simulink model "Tank1"  (R2023a)
settings: Solver=VariableStepAuto  StartTime=0.0  StopTime=100  RelTol=1e-3
settings Model: Creator=hch  LastModifiedBy=hch

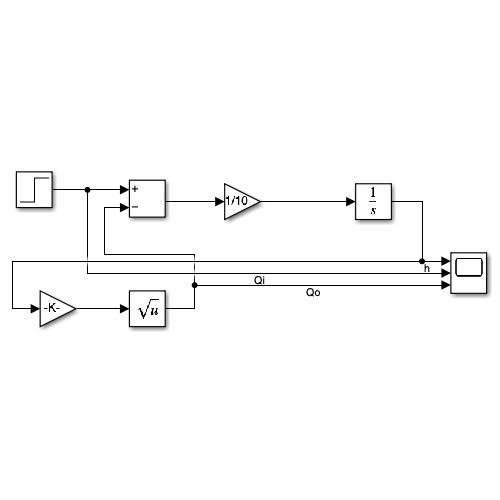
[thumbnail: Simulink's stored preview of the top-level diagram]
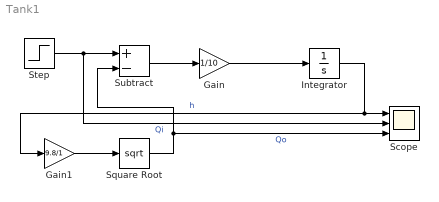
== system Tank1 ==
  Gain : Gain  Gain=1/10
  Gain1 : Gain  Gain=9.8/1
  Integrator : Integrator  InitialCondition=10
  Scope : Scope  NumInputPorts=3
  Square Root : Sqrt
  Step : Step  Time=0  Before=0.03  After=0.03  SampleTime=0
  Subtract : Sum  Inputs=+-
  wires:
  Subtract/1 -> Gain/1
  Step/1 -> Scope/2, Subtract/1  "Qi"
  Gain/1 -> Integrator/1
  Gain1/1 -> Square Root/1
  Integrator/1 -> Scope/1, Gain1/1  "h"
  Square Root/1 -> Scope/3, Subtract/2  "Qo"
